simulink model "CW_m26"  (R2020b)
settings: Solver=ode3  StartTime=0.0  StopTime=simTime  FixedStep=0.001  RelTol=1e-3  EnableMultiTasking=on
undefined symbols (not defined in the file): b, J, K, L, R
settings Model: Creator=aarrieta  LastModifiedBy=Xiao Ling
settings DataIOCC: ExternalInput=var  SaveFormat=Array  SignalLogging=off  DSMLogging=off  ReturnWorkspaceOutputs=off
settings OptimizationCC: LifeSpan=inf
settings DebuggingCC: UnderspecifiedInitializationDetection=Classic  MergeDetectMultiDrivingBlocksExec=none  SolverPrmCheckMsg=warning  StateNameClashWarn=warning  SFUnexpectedBacktrackingDiag=warning  SFNoUnconditionalDefaultTransitionDiag=warning  SFExecutionAtInitializationDiag=none  ArithmeticOperatorsInVariantConditions=warning
settings HardwareCC: ProdBitPerPointer=32  ProdBitPerSizeT=32  ProdBitPerPtrDiffT=32  ProdLargestAtomicFloat=None  ProdIntDivRoundTo=Undefined  ProdEndianess=Unspecified  ProdWordSize=32  ProdHWDeviceType=32-bit Generic
settings ModelReferenceCC: PropagateSignalLabelsOutOfModel=off
settings SFSimCC: SimUseLocalCustomCode=off  CustomCodeUndefinedFunction=UseInterfaceOnly
settings RTWCC: RTWUseLocalCustomCode=off
settings CodeAppCC: StateflowObjectComments=on
settings GRTTargetCC: TargetLangStandard=C89/C90 (ANSI)
settings ConfigComp: CovScope=ReferencedModels  CovMetricSettings=dcmtw  CovHTMLOptions=-sRT=1 -aTS=1 -bRG=1 -bTC=1 -hTR=0 -nFC=0 -scm=1 -bcm=1 -xEv=0  CovSaveCumulativeToWorkspaceVar=on  CovSaveSingleToWorkspaceVar=on  DVMaxTestCaseSteps=500  DVTestSuiteOptimization=CombinedObjectives (Nonlinear Extended)  DVDetectActiveLogic=on
settings SimscapeCC: SimscapeNormalizeSystem=off
settings ConfigurationSet: Description=SimMechanics 2G

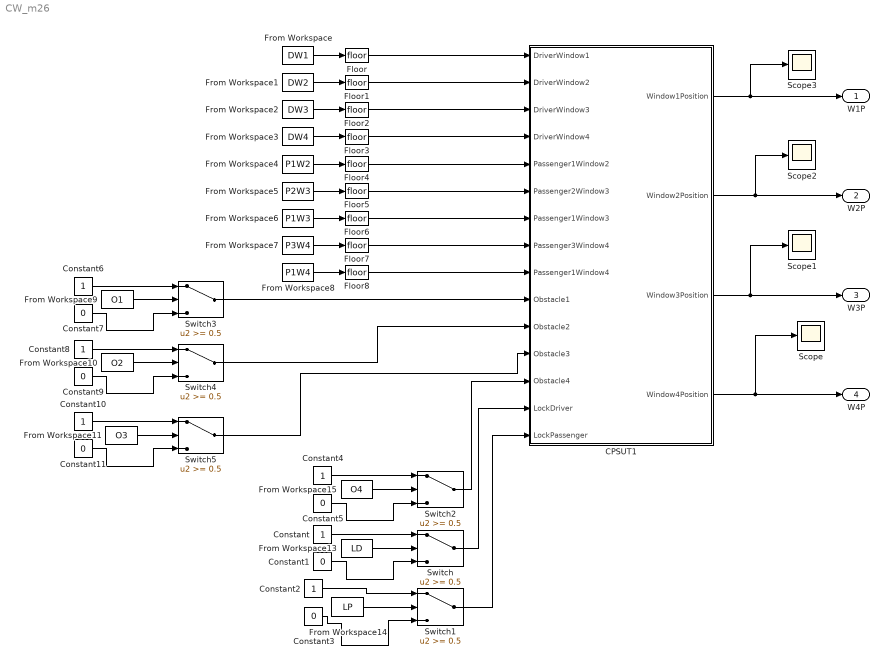
== system CW_m26 ==
  CPSUT1 : Subsystem
  Constant{,2,4,6,8,10} (6 alike) : Constant  OutDataTypeStr=boolean
  Constant{1,3,5,7,9,11} (6 alike) : Constant  Value=0  OutDataTypeStr=boolean
  Floor{,1..8} (9 alike) : Rounding
  From Workspace : FromWorkspace  VariableName=DW1
  From Workspace1 : FromWorkspace  VariableName=DW2
  From Workspace10 : FromWorkspace  VariableName=O2
  From Workspace11 : FromWorkspace  VariableName=O3
  From Workspace13 : FromWorkspace  VariableName=LD
  From Workspace14 : FromWorkspace  VariableName=LP
  From Workspace15 : FromWorkspace  VariableName=O4
  From Workspace2 : FromWorkspace  VariableName=DW3
  From Workspace3 : FromWorkspace  VariableName=DW4
  From Workspace4 : FromWorkspace  VariableName=P1W2
  From Workspace5 : FromWorkspace  VariableName=P2W3
  From Workspace6 : FromWorkspace  VariableName=P1W3
  From Workspace7 : FromWorkspace  VariableName=P3W4
  From Workspace8 : FromWorkspace  VariableName=P1W4
  From Workspace9 : FromWorkspace  VariableName=O1
  Scope{,1..3} (4 alike) : Scope
  Switch{,1..5} (6 alike) : Switch  Threshold=0.5
  W1P : Outport
  W2P : Outport  Port=2
  W3P : Outport  Port=3
  W4P : Outport  Port=4
  wires:
  CPSUT1/1(Window1Position) -> W1P/1, Scope3/1
  CPSUT1/2(Window2Position) -> W2P/1, Scope2/1
  CPSUT1/3(Window3Position) -> W3P/1, Scope1/1
  CPSUT1/4(Window4Position) -> W4P/1, Scope/1
  From Workspace2/1 -> Floor2/1
  From Workspace3/1 -> Floor3/1
  From Workspace4/1 -> Floor4/1
  From Workspace5/1 -> Floor5/1
  From Workspace6/1 -> Floor6/1
  From Workspace7/1 -> Floor7/1
  From Workspace8/1 -> Floor8/1
  Switch2/1 -> CPSUT1/13(Obstacle4)
  From Workspace13/1 -> Switch/2
  From Workspace14/1 -> Switch1/2
  Switch1/1 -> CPSUT1/15(LockPassenger)
  Constant/1 -> Switch/1
  Constant1/1 -> Switch/3
  Constant2/1 -> Switch1/1
  Constant3/1 -> Switch1/3
  Switch/1 -> CPSUT1/14(LockDriver)
  From Workspace/1 -> Floor/1
  Floor/1 -> CPSUT1/1(DriverWindow1)
  From Workspace1/1 -> Floor1/1
  Floor1/1 -> CPSUT1/2(DriverWindow2)
  Floor2/1 -> CPSUT1/3(DriverWindow3)
  Floor3/1 -> CPSUT1/4(DriverWindow4)
  Floor4/1 -> CPSUT1/5(Passenger1Window2)
  Floor5/1 -> CPSUT1/6(Passenger2Window3)
  Floor6/1 -> CPSUT1/7(Passenger1Window3)
  Floor7/1 -> CPSUT1/8(Passenger3Window4)
  Floor8/1 -> CPSUT1/9(Passenger1Window4)
  From Workspace15/1 -> Switch2/2
  Constant5/1 -> Switch2/3
  Constant4/1 -> Switch2/1
  Constant7/1 -> Switch3/3
  From Workspace9/1 -> Switch3/2
  Switch3/1 -> CPSUT1/10(Obstacle1)
  Constant6/1 -> Switch3/1
  Constant9/1 -> Switch4/3
  From Workspace10/1 -> Switch4/2
  Switch4/1 -> CPSUT1/11(Obstacle2)
  Constant8/1 -> Switch4/1
  Constant11/1 -> Switch5/3
  From Workspace11/1 -> Switch5/2
  Switch5/1 -> CPSUT1/12(Obstacle3)
  Constant10/1 -> Switch5/1

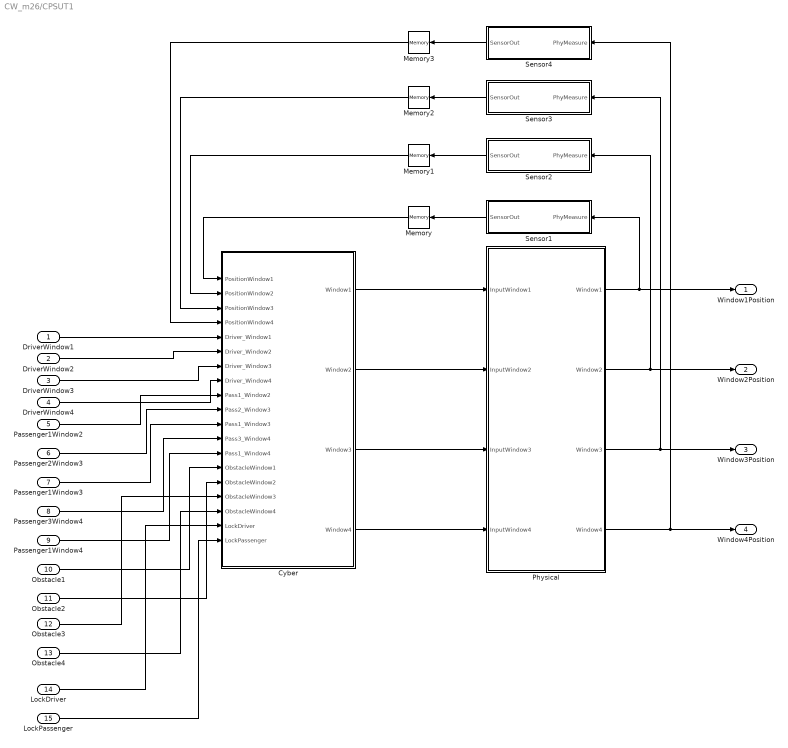
== system CW_m26/CPSUT1 ==
  DriverWindow1 : Inport
  DriverWindow2 : Inport  Port=2
  DriverWindow3 : Inport  Port=3
  DriverWindow4 : Inport  Port=4
  Passenger1Window2 : Inport  Port=5
  Passenger2Window3 : Inport  Port=6
  Passenger1Window3 : Inport  Port=7
  Passenger3Window4 : Inport  Port=8
  Passenger1Window4 : Inport  Port=9
  Obstacle1 : Inport  Port=10
  Obstacle2 : Inport  Port=11
  Obstacle3 : Inport  Port=12
  Obstacle4 : Inport  Port=13
  LockDriver : Inport  Port=14
  LockPassenger : Inport  Port=15
  Cyber : Subsystem
  Memory{,1..3} (4 alike) : Memory
  Physical : Subsystem
  Sensor1 : Subsystem
  Sensor2 : Subsystem
  Sensor3 : Subsystem
  Sensor4 : Subsystem
  Window1Position : Outport  VectorParamsAs1DForOutWhenUnconnected=off
  Window2Position : Outport  Port=2  VectorParamsAs1DForOutWhenUnconnected=off
  Window3Position : Outport  Port=3  VectorParamsAs1DForOutWhenUnconnected=off
  Window4Position : Outport  Port=4  VectorParamsAs1DForOutWhenUnconnected=off
  wires:
  Cyber/4(Window4) -> Physical/4(InputWindow4)
  Cyber/3(Window3) -> Physical/3(InputWindow3)
  Cyber/2(Window2) -> Physical/2(InputWindow2)
  Cyber/1(Window1) -> Physical/1(InputWindow1)
  Physical/1(Window1) -> Sensor1/1(PhyMeasure), Window1Position/1
  Physical/2(Window2) -> Sensor2/1(PhyMeasure), Window2Position/1
  Physical/3(Window3) -> Window3Position/1, Sensor3/1(PhyMeasure)
  Physical/4(Window4) -> Sensor4/1(PhyMeasure), Window4Position/1
  Memory/1 -> Cyber/1(PositionWindow1)
  Memory1/1 -> Cyber/2(PositionWindow2)
  Memory2/1 -> Cyber/3(PositionWindow3)
  Memory3/1 -> Cyber/4(PositionWindow4)
  Obstacle1/1 -> Cyber/14(ObstacleWindow1)
  Sensor4/1(SensorOut) -> Memory3/1
  Sensor3/1(SensorOut) -> Memory2/1
  Sensor2/1(SensorOut) -> Memory1/1
  Sensor1/1(SensorOut) -> Memory/1
  DriverWindow2/1 -> Cyber/6(Driver_Window2)
  DriverWindow1/1 -> Cyber/5(Driver_Window1)
  DriverWindow3/1 -> Cyber/7(Driver_Window3)
  DriverWindow4/1 -> Cyber/8(Driver_Window4)
  Passenger1Window2/1 -> Cyber/9(Pass1_Window2)
  Passenger2Window3/1 -> Cyber/10(Pass2_Window3)
  Passenger1Window3/1 -> Cyber/11(Pass1_Window3)
  Passenger3Window4/1 -> Cyber/12(Pass3_Window4)
  Passenger1Window4/1 -> Cyber/13(Pass1_Window4)
  Obstacle2/1 -> Cyber/15(ObstacleWindow2)
  Obstacle3/1 -> Cyber/16(ObstacleWindow3)
  Obstacle4/1 -> Cyber/17(ObstacleWindow4)
  LockDriver/1 -> Cyber/18(LockDriver)
  LockPassenger/1 -> Cyber/19(LockPassenger)

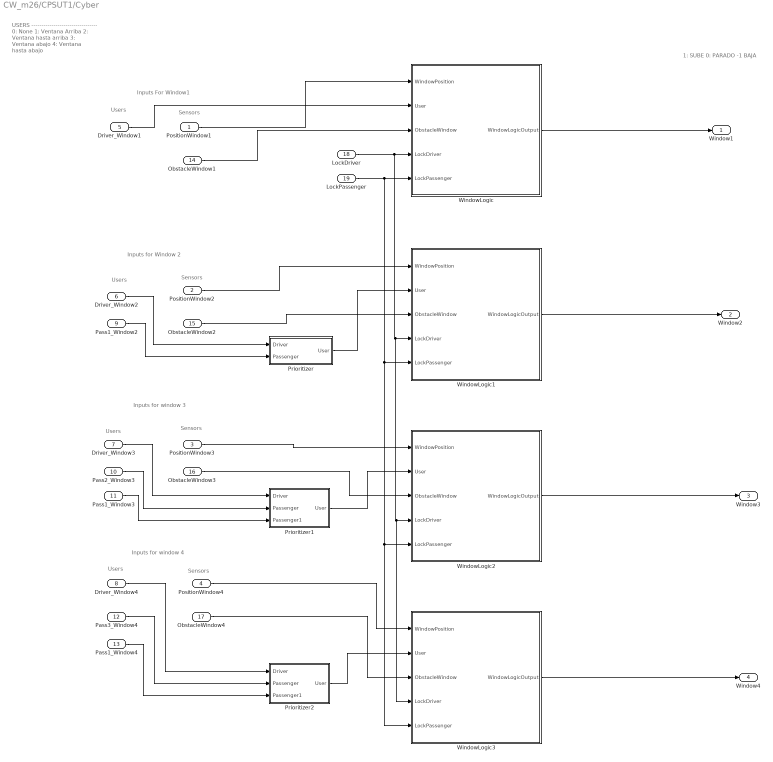
== system CW_m26/CPSUT1/Cyber ==
  note: 1: SUBE
      | 0: PARADO
      | -1 BAJA
  note: USERS
      | ---------------------------------
      | 0: None
      | 1: Ventana Arriba
      | 2: Ventana hasta arriba
      | 3: Ventana abajo
      | 4: Ventana hasta abajo
  note: Sensors
  note: Users
  note: Sensors
  note: Users
  note: Sensors
  note: Users
  note: Users
  note: Sensors
  note: Inputs for window 4
  note: Inputs for window 3
  note: Inputs for Window 2
  note: Inputs For Window1
  PositionWindow1 : Inport
  PositionWindow2 : Inport  Port=2
  PositionWindow3 : Inport  Port=3
  PositionWindow4 : Inport  Port=4
  Driver_Window1 : Inport  Port=5
  Driver_Window2 : Inport  Port=6
  Driver_Window3 : Inport  Port=7
  Driver_Window4 : Inport  Port=8
  Pass1_Window2 : Inport  Port=9
  Pass2_Window3 : Inport  Port=10
  Pass1_Window3 : Inport  Port=11
  Pass3_Window4 : Inport  Port=12
  Pass1_Window4 : Inport  Port=13
  ObstacleWindow1 : Inport  Port=14
  ObstacleWindow2 : Inport  Port=15
  ObstacleWindow3 : Inport  Port=16
  ObstacleWindow4 : Inport  Port=17
  LockDriver : Inport  Port=18
  LockPassenger : Inport  Port=19
  Prioritizer : Subsystem
  Prioritizer1 : Subsystem
  Prioritizer2 : Subsystem
  WindowLogic : Subsystem
  WindowLogic1 : Subsystem
  WindowLogic2 : Subsystem
  WindowLogic3 : Subsystem
  Window1 : Outport  VectorParamsAs1DForOutWhenUnconnected=off
  Window2 : Outport  Port=2  VectorParamsAs1DForOutWhenUnconnected=off
  Window3 : Outport  Port=3  VectorParamsAs1DForOutWhenUnconnected=off
  Window4 : Outport  Port=4  VectorParamsAs1DForOutWhenUnconnected=off
  wires:
  LockDriver/1 -> WindowLogic1/4(LockDriver), WindowLogic3/4(LockDriver), WindowLogic2/4(LockDriver), WindowLogic/4(LockDriver)
  LockPassenger/1 -> WindowLogic1/5(LockPassenger), WindowLogic3/5(LockPassenger), WindowLogic2/5(LockPassenger), WindowLogic/5(LockPassenger)
  PositionWindow1/1 -> WindowLogic/1(WindowPosition)
  ObstacleWindow1/1 -> WindowLogic/3(ObstacleWindow)
  Driver_Window1/1 -> WindowLogic/2(User)
  WindowLogic/1(WindowLogicOutput) -> Window1/1
  Prioritizer/1(User) -> WindowLogic1/2(User)
  Driver_Window2/1 -> Prioritizer/1(Driver)
  Pass1_Window2/1 -> Prioritizer/2(Passenger)
  PositionWindow2/1 -> WindowLogic1/1(WindowPosition)
  ObstacleWindow2/1 -> WindowLogic1/3(ObstacleWindow)
  WindowLogic1/1(WindowLogicOutput) -> Window2/1
  Prioritizer1/1(User) -> WindowLogic2/2(User)
  PositionWindow3/1 -> WindowLogic2/1(WindowPosition)
  ObstacleWindow3/1 -> WindowLogic2/3(ObstacleWindow)
  Driver_Window3/1 -> Prioritizer1/1(Driver)
  Pass2_Window3/1 -> Prioritizer1/2(Passenger)
  Pass1_Window3/1 -> Prioritizer1/3(Passenger1)
  Driver_Window4/1 -> Prioritizer2/1(Driver)
  Pass3_Window4/1 -> Prioritizer2/2(Passenger)
  Pass1_Window4/1 -> Prioritizer2/3(Passenger1)
  PositionWindow4/1 -> WindowLogic3/1(WindowPosition)
  ObstacleWindow4/1 -> WindowLogic3/3(ObstacleWindow)
  Prioritizer2/1(User) -> WindowLogic3/2(User)
  WindowLogic2/1(WindowLogicOutput) -> Window3/1
  WindowLogic3/1(WindowLogicOutput) -> Window4/1

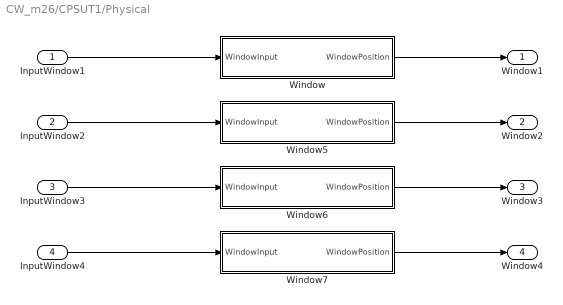
== system CW_m26/CPSUT1/Physical ==
  InputWindow1 : Inport
  InputWindow2 : Inport  Port=2
  InputWindow3 : Inport  Port=3
  InputWindow4 : Inport  Port=4
  Window : Subsystem
  Window5 : Subsystem
  Window6 : Subsystem
  Window7 : Subsystem
  Window1 : Outport  VectorParamsAs1DForOutWhenUnconnected=off
  Window2 : Outport  Port=2  VectorParamsAs1DForOutWhenUnconnected=off
  Window3 : Outport  Port=3  VectorParamsAs1DForOutWhenUnconnected=off
  Window4 : Outport  Port=4  VectorParamsAs1DForOutWhenUnconnected=off
  wires:
  InputWindow1/1 -> Window/1(WindowInput)
  InputWindow2/1 -> Window5/1(WindowInput)
  InputWindow3/1 -> Window6/1(WindowInput)
  InputWindow4/1 -> Window7/1(WindowInput)
  Window/1(WindowPosition) -> Window1/1
  Window5/1(WindowPosition) -> Window2/1
  Window6/1(WindowPosition) -> Window3/1
  Window7/1(WindowPosition) -> Window4/1

== system CW_m26/CPSUT1/Sensor1 ==
  PhyMeasure : Inport
  SensorOut : Outport  VectorParamsAs1DForOutWhenUnconnected=off
  wires:
  PhyMeasure/1 -> SensorOut/1

== system CW_m26/CPSUT1/Sensor2 ==
  PhyMeasure : Inport
  SensorOut : Outport  VectorParamsAs1DForOutWhenUnconnected=off
  wires:
  PhyMeasure/1 -> SensorOut/1

== system CW_m26/CPSUT1/Sensor3 ==
  PhyMeasure : Inport
  SensorOut : Outport  VectorParamsAs1DForOutWhenUnconnected=off
  wires:
  PhyMeasure/1 -> SensorOut/1

== system CW_m26/CPSUT1/Sensor4 ==
  PhyMeasure : Inport
  SensorOut : Outport  VectorParamsAs1DForOutWhenUnconnected=off
  wires:
  PhyMeasure/1 -> SensorOut/1

== system CW_m26/CPSUT1/Cyber/Prioritizer ==
  Driver : Inport
  Passenger : Inport  Port=2
  Switch : Switch  Criteria=u2 ~= 0
  User : Outport  VectorParamsAs1DForOutWhenUnconnected=off
  wires:
  Driver/1 -> Switch/1, Switch/2
  Passenger/1 -> Switch/3
  Switch/1 -> User/1

== system CW_m26/CPSUT1/Cyber/Prioritizer1 ==
  Driver : Inport
  Passenger : Inport  Port=2
  Passenger1 : Inport  Port=3
  Switch : Switch  Criteria=u2 ~= 0
  Switch1 : Switch  Criteria=u2 ~= 0
  User : Outport  VectorParamsAs1DForOutWhenUnconnected=off
  wires:
  Switch/1 -> User/1
  Passenger/1 -> Switch1/1, Switch1/2
  Driver/1 -> Switch/1, Switch/2
  Passenger1/1 -> Switch1/3
  Switch1/1 -> Switch/3

== system CW_m26/CPSUT1/Cyber/Prioritizer2 ==
  Driver : Inport
  Passenger : Inport  Port=2
  Passenger1 : Inport  Port=3
  Switch : Switch  Criteria=u2 ~= 0
  Switch1 : Switch  Criteria=u2 ~= 0
  User : Outport  VectorParamsAs1DForOutWhenUnconnected=off
  wires:
  Switch1/1 -> Switch/3
  Passenger1/1 -> Switch1/3
  Driver/1 -> Switch/2, Switch/1
  Passenger/1 -> Switch1/2, Switch1/1
  Switch/1 -> User/1

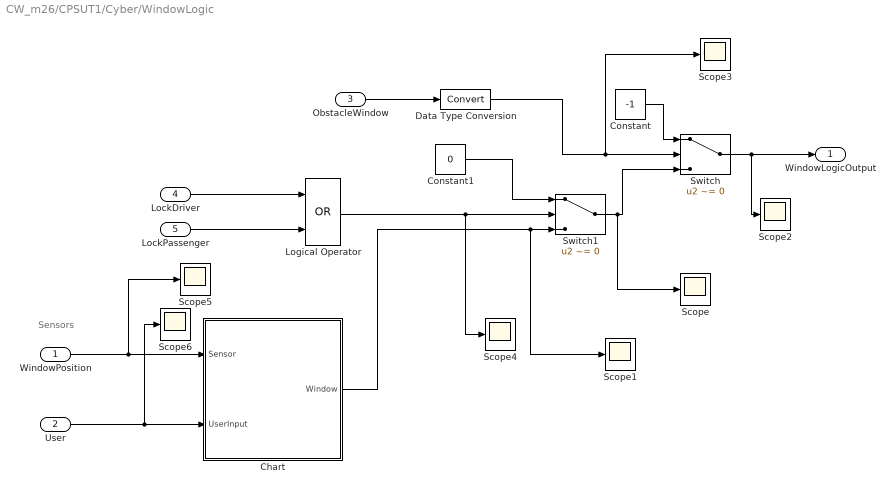
== system CW_m26/CPSUT1/Cyber/WindowLogic ==
  note: Sensors
  WindowPosition : Inport
  User : Inport  Port=2
  ObstacleWindow : Inport  Port=3
  LockDriver : Inport  Port=4
  LockPassenger : Inport  Port=5
  Chart : Stateflow chart  TreatAsAtomicUnit=on
  Constant : Constant  Value=-1
  Constant1 : Constant  Value=0
  Data Type Conversion : DataTypeConversion
  Logical Operator : Logic  Operator=OR  AllPortsSameDT=off  OutDataTypeStr=boolean
  Scope{,1..6} (7 alike) : Scope
  Switch : Switch  Criteria=u2 ~= 0  Threshold=1  ZeroCross=off
  Switch1 : Switch  Criteria=u2 ~= 0
  WindowLogicOutput : Outport  VectorParamsAs1DForOutWhenUnconnected=off
  wires:
  LockDriver/1 -> Logical Operator/1
  LockPassenger/1 -> Logical Operator/2
  ObstacleWindow/1 -> Data Type Conversion/1
  Switch/1 -> Scope2/1, WindowLogicOutput/1
  Constant1/1 -> Switch1/1
  Switch1/1 -> Scope/1, Switch/3
  WindowPosition/1 -> Scope5/1, Chart/1(Sensor)
  User/1 -> Chart/2(UserInput), Scope6/1
  Chart/1(Window) -> Scope1/1, Switch1/3
  Constant/1 -> Switch/1
  Data Type Conversion/1 -> Scope3/1, Switch/2
  Logical Operator/1 -> Scope4/1, Switch1/2

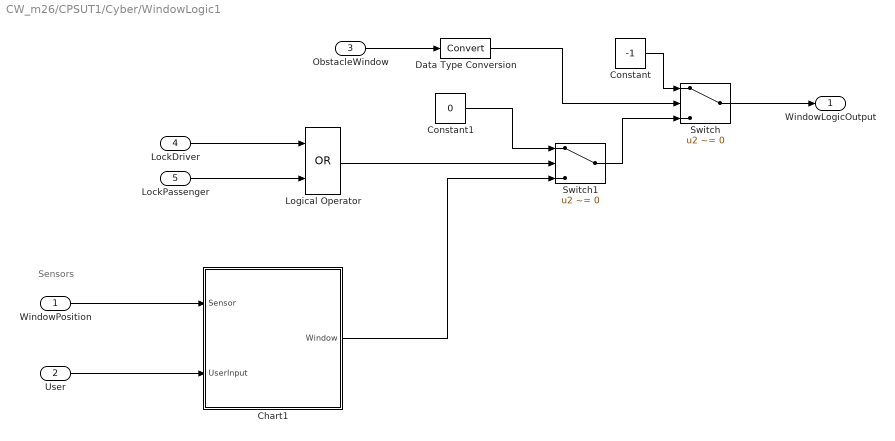
== system CW_m26/CPSUT1/Cyber/WindowLogic1 ==
  note: Sensors
  WindowPosition : Inport
  User : Inport  Port=2
  ObstacleWindow : Inport  Port=3
  LockDriver : Inport  Port=4
  LockPassenger : Inport  Port=5
  Chart1 : Stateflow chart  TreatAsAtomicUnit=on
  Constant : Constant  Value=-1
  Constant1 : Constant  Value=0
  Data Type Conversion : DataTypeConversion
  Logical Operator : Logic  Operator=OR  AllPortsSameDT=off  OutDataTypeStr=boolean
  Switch : Switch  Criteria=u2 ~= 0  Threshold=1  ZeroCross=off
  Switch1 : Switch  Criteria=u2 ~= 0
  WindowLogicOutput : Outport  VectorParamsAs1DForOutWhenUnconnected=off
  wires:
  Logical Operator/1 -> Switch1/2
  Data Type Conversion/1 -> Switch/2
  Constant/1 -> Switch/1
  Chart1/1(Window) -> Switch1/3
  User/1 -> Chart1/2(UserInput)
  WindowPosition/1 -> Chart1/1(Sensor)
  Switch1/1 -> Switch/3
  Constant1/1 -> Switch1/1
  Switch/1 -> WindowLogicOutput/1
  ObstacleWindow/1 -> Data Type Conversion/1
  LockPassenger/1 -> Logical Operator/2
  LockDriver/1 -> Logical Operator/1

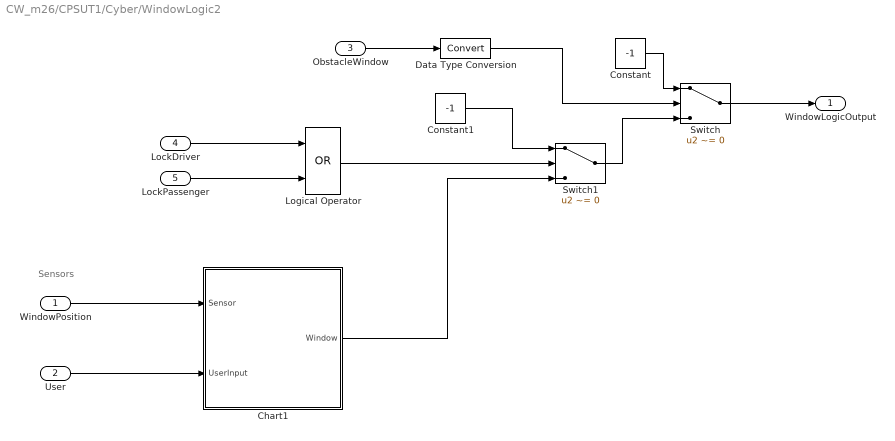
== system CW_m26/CPSUT1/Cyber/WindowLogic2 ==
  note: Sensors
  WindowPosition : Inport
  User : Inport  Port=2
  ObstacleWindow : Inport  Port=3
  LockDriver : Inport  Port=4
  LockPassenger : Inport  Port=5
  Chart1 : Stateflow chart  TreatAsAtomicUnit=on
  Constant : Constant  Value=-1
  Constant1 : Constant  Value=-1
  Data Type Conversion : DataTypeConversion
  Logical Operator : Logic  Operator=OR  AllPortsSameDT=off  OutDataTypeStr=boolean
  Switch : Switch  Criteria=u2 ~= 0  Threshold=1  ZeroCross=off
  Switch1 : Switch  Criteria=u2 ~= 0
  WindowLogicOutput : Outport  VectorParamsAs1DForOutWhenUnconnected=off
  wires:
  LockDriver/1 -> Logical Operator/1
  LockPassenger/1 -> Logical Operator/2
  ObstacleWindow/1 -> Data Type Conversion/1
  Switch/1 -> WindowLogicOutput/1
  Constant1/1 -> Switch1/1
  Switch1/1 -> Switch/3
  WindowPosition/1 -> Chart1/1(Sensor)
  User/1 -> Chart1/2(UserInput)
  Chart1/1(Window) -> Switch1/3
  Constant/1 -> Switch/1
  Data Type Conversion/1 -> Switch/2
  Logical Operator/1 -> Switch1/2

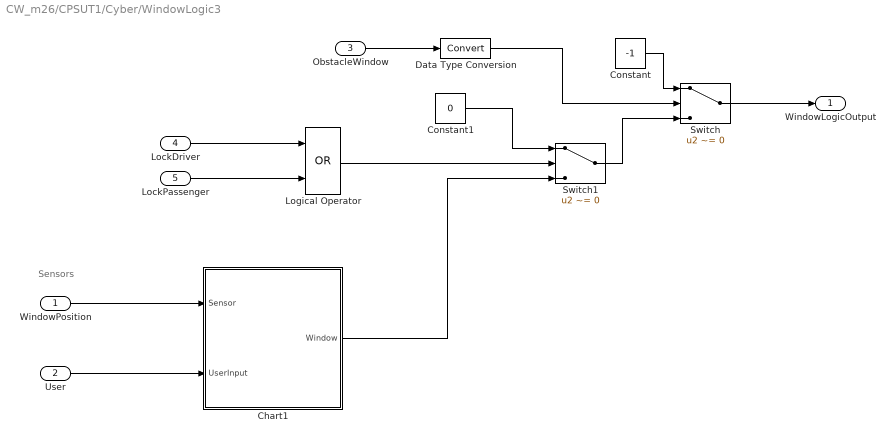
== system CW_m26/CPSUT1/Cyber/WindowLogic3 ==
  note: Sensors
  WindowPosition : Inport
  User : Inport  Port=2
  ObstacleWindow : Inport  Port=3
  LockDriver : Inport  Port=4
  LockPassenger : Inport  Port=5
  Chart1 : Stateflow chart  TreatAsAtomicUnit=on
  Constant : Constant  Value=-1
  Constant1 : Constant  Value=0
  Data Type Conversion : DataTypeConversion
  Logical Operator : Logic  Operator=OR  AllPortsSameDT=off  OutDataTypeStr=boolean
  Switch : Switch  Criteria=u2 ~= 0  Threshold=1  ZeroCross=off
  Switch1 : Switch  Criteria=u2 ~= 0
  WindowLogicOutput : Outport  VectorParamsAs1DForOutWhenUnconnected=off
  wires:
  Logical Operator/1 -> Switch1/2
  Data Type Conversion/1 -> Switch/2
  Constant/1 -> Switch/1
  Chart1/1(Window) -> Switch1/3
  User/1 -> Chart1/2(UserInput)
  WindowPosition/1 -> Chart1/1(Sensor)
  Switch1/1 -> Switch/3
  Constant1/1 -> Switch1/1
  Switch/1 -> WindowLogicOutput/1
  ObstacleWindow/1 -> Data Type Conversion/1
  LockPassenger/1 -> Logical Operator/2
  LockDriver/1 -> Logical Operator/1

== system CW_m26/CPSUT1/Physical/Window ==
  WindowInput : Inport
  DC_Engine : Subsystem
  Integrator : Integrator  InitialCondition=5  LimitOutput=on  UpperSaturationLimit=5  LowerSaturationLimit=0
  WindowPosition : Outport  VectorParamsAs1DForOutWhenUnconnected=off
  wires:
  Integrator/1 -> WindowPosition/1
  DC_Engine/1(Speed) -> Integrator/1
  WindowInput/1 -> DC_Engine/1(input)

== system CW_m26/CPSUT1/Physical/Window5 ==
  WindowInput : Inport
  DC_Engine : Subsystem
  Integrator : Integrator  InitialCondition=5  LimitOutput=on  UpperSaturationLimit=5  LowerSaturationLimit=0
  WindowPosition : Outport  VectorParamsAs1DForOutWhenUnconnected=off
  wires:
  WindowInput/1 -> DC_Engine/1(input)
  DC_Engine/1(Speed) -> Integrator/1
  Integrator/1 -> WindowPosition/1

== system CW_m26/CPSUT1/Physical/Window6 ==
  WindowInput : Inport
  DC_Engine : Subsystem
  Integrator : Integrator  InitialCondition=5  LimitOutput=on  UpperSaturationLimit=5  LowerSaturationLimit=0
  WindowPosition : Outport  VectorParamsAs1DForOutWhenUnconnected=off
  wires:
  Integrator/1 -> WindowPosition/1
  DC_Engine/1(Speed) -> Integrator/1
  WindowInput/1 -> DC_Engine/1(input)

== system CW_m26/CPSUT1/Physical/Window7 ==
  WindowInput : Inport
  DC_Engine : Subsystem
  Integrator : Integrator  InitialCondition=5  LimitOutput=on  UpperSaturationLimit=5  LowerSaturationLimit=0
  WindowPosition : Outport  VectorParamsAs1DForOutWhenUnconnected=off
  wires:
  WindowInput/1 -> DC_Engine/1(input)
  DC_Engine/1(Speed) -> Integrator/1
  Integrator/1 -> WindowPosition/1

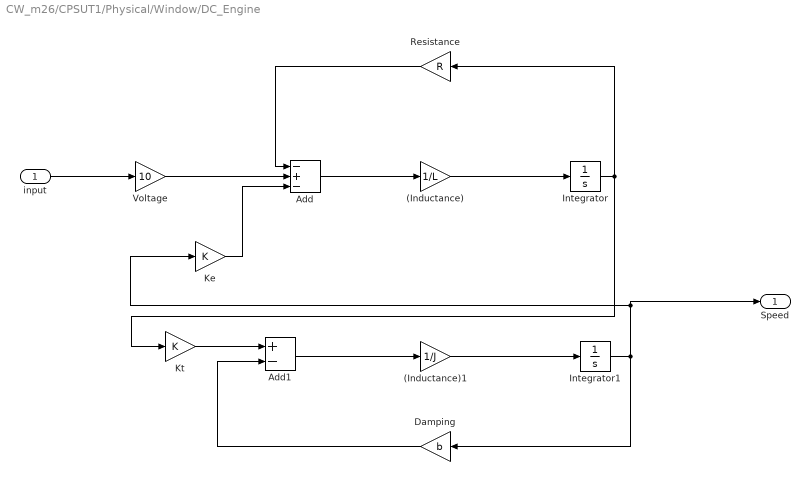
== system CW_m26/CPSUT1/Physical/Window/DC_Engine ==
  input : Inport
  (Inductance) : Gain  Gain=1/L
  (Inductance)1 : Gain  Gain=1/J
  Add : Sum  Inputs=-+-
  Add1 : Sum  Inputs=+-
  Damping : Gain  Gain=b
  Integrator : Integrator
  Integrator1 : Integrator
  Ke : Gain  Gain=K
  Kt : Gain  Gain=K
  Resistance : Gain  Gain=R
  Voltage : Gain  Gain=10
  Speed : Outport  VectorParamsAs1DForOutWhenUnconnected=off
  wires:
  input/1 -> Voltage/1
  Voltage/1 -> Add/2
  Add/1 -> (Inductance)/1
  (Inductance)/1 -> Integrator/1
  Integrator/1 -> Kt/1, Resistance/1
  Resistance/1 -> Add/1
  Ke/1 -> Add/3
  Kt/1 -> Add1/1
  Add1/1 -> (Inductance)1/1
  (Inductance)1/1 -> Integrator1/1
  Integrator1/1 -> Ke/1, Speed/1, Damping/1
  Damping/1 -> Add1/2

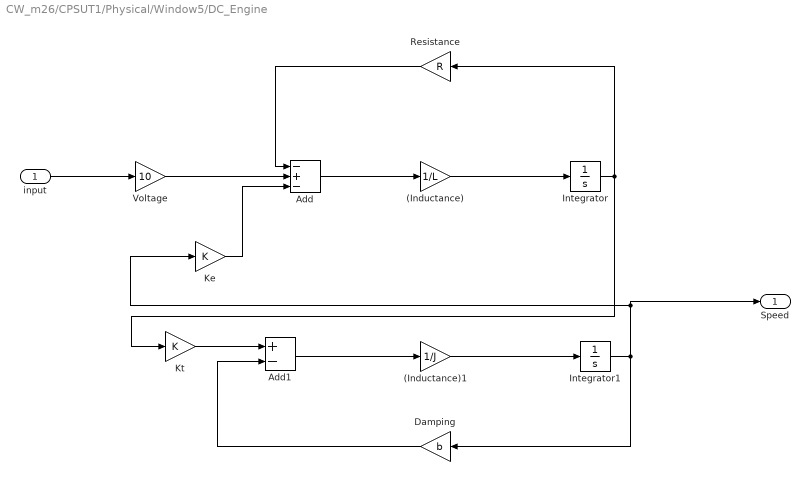
== system CW_m26/CPSUT1/Physical/Window5/DC_Engine ==
  input : Inport
  (Inductance) : Gain  Gain=1/L
  (Inductance)1 : Gain  Gain=1/J
  Add : Sum  Inputs=-+-
  Add1 : Sum  Inputs=+-
  Damping : Gain  Gain=b
  Integrator : Integrator
  Integrator1 : Integrator
  Ke : Gain  Gain=K
  Kt : Gain  Gain=K
  Resistance : Gain  Gain=R
  Voltage : Gain  Gain=10
  Speed : Outport  VectorParamsAs1DForOutWhenUnconnected=off
  wires:
  Damping/1 -> Add1/2
  Integrator1/1 -> Damping/1, Speed/1, Ke/1
  (Inductance)1/1 -> Integrator1/1
  Add1/1 -> (Inductance)1/1
  Kt/1 -> Add1/1
  Ke/1 -> Add/3
  Resistance/1 -> Add/1
  Integrator/1 -> Resistance/1, Kt/1
  (Inductance)/1 -> Integrator/1
  Add/1 -> (Inductance)/1
  Voltage/1 -> Add/2
  input/1 -> Voltage/1

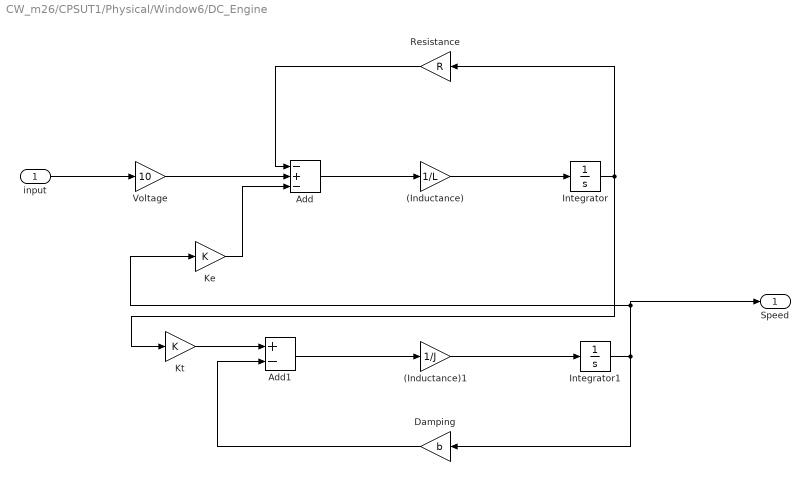
== system CW_m26/CPSUT1/Physical/Window6/DC_Engine ==
  input : Inport
  (Inductance) : Gain  Gain=1/L
  (Inductance)1 : Gain  Gain=1/J
  Add : Sum  Inputs=-+-
  Add1 : Sum  Inputs=+-
  Damping : Gain  Gain=b
  Integrator : Integrator
  Integrator1 : Integrator
  Ke : Gain  Gain=K
  Kt : Gain  Gain=K
  Resistance : Gain  Gain=R
  Voltage : Gain  Gain=10
  Speed : Outport  VectorParamsAs1DForOutWhenUnconnected=off
  wires:
  input/1 -> Voltage/1
  Voltage/1 -> Add/2
  Add/1 -> (Inductance)/1
  (Inductance)/1 -> Integrator/1
  Integrator/1 -> Kt/1, Resistance/1
  Resistance/1 -> Add/1
  Ke/1 -> Add/3
  Kt/1 -> Add1/1
  Add1/1 -> (Inductance)1/1
  (Inductance)1/1 -> Integrator1/1
  Integrator1/1 -> Ke/1, Speed/1, Damping/1
  Damping/1 -> Add1/2

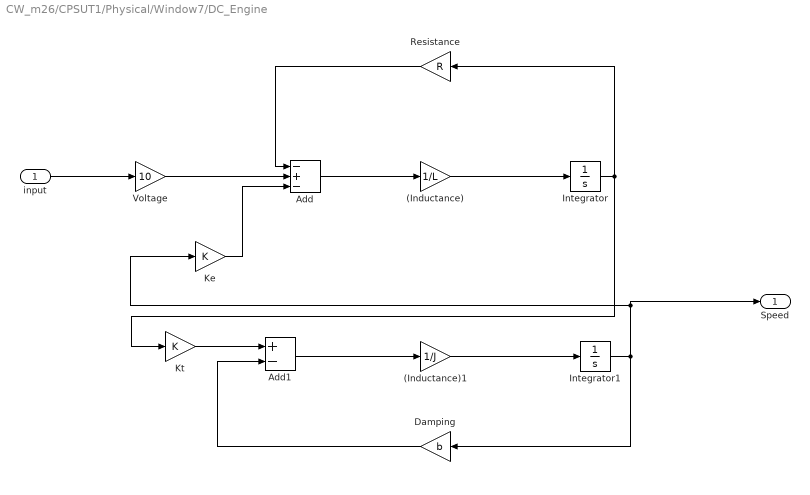
== system CW_m26/CPSUT1/Physical/Window7/DC_Engine ==
  input : Inport
  (Inductance) : Gain  Gain=1/L
  (Inductance)1 : Gain  Gain=1/J
  Add : Sum  Inputs=-+-
  Add1 : Sum  Inputs=+-
  Damping : Gain  Gain=b
  Integrator : Integrator
  Integrator1 : Integrator
  Ke : Gain  Gain=K
  Kt : Gain  Gain=K
  Resistance : Gain  Gain=R
  Voltage : Gain  Gain=10
  Speed : Outport  VectorParamsAs1DForOutWhenUnconnected=off
  wires:
  Damping/1 -> Add1/2
  Integrator1/1 -> Damping/1, Speed/1, Ke/1
  (Inductance)1/1 -> Integrator1/1
  Add1/1 -> (Inductance)1/1
  Kt/1 -> Add1/1
  Ke/1 -> Add/3
  Resistance/1 -> Add/1
  Integrator/1 -> Resistance/1, Kt/1
  (Inductance)/1 -> Integrator/1
  Add/1 -> (Inductance)/1
  Voltage/1 -> Add/2
  input/1 -> Voltage/1

== stateflow chart CW_m26/CPSUT1/Cyber/WindowLogic1/Chart1 ==
  state Bajand_hasta_abajo
    entry: Window = -1;
  state Bajando
    entry: Window = -1;
  state Idle
    entry:Window = 0;
  state Subiendo_hasta_arriba
    entry: Window = 1;
  state Subiendo
    entry: Window = 1;
  Subiendo -> Bajand_hasta_abajo [order 4] : [UserInput==4]
  Bajand_hasta_abajo -> Bajando [order 2] : [UserInput==3]
  Subiendo -> Bajando [order 3] : [UserInput==3]
  Bajando -> Bajand_hasta_abajo [order 2] : [UserInput==4]
  Idle -> Bajando [order 3] : [UserInput==3&&Sensor>0]
  Subiendo_hasta_arriba -> Bajand_hasta_abajo [order 3] : [UserInput==4]
  Idle -> Bajand_hasta_abajo [order 4] : [UserInput==4&&Sensor>0]
  Bajando -> Subiendo [order 3] : [UserInput==1]
  Subiendo_hasta_arriba -> Bajando [order 4] : [UserInput==3]
  Bajand_hasta_abajo -> Subiendo [order 4] : [UserInput==1]
  Bajand_hasta_abajo -> Idle [order 1] : [Sensor<=0]
  Bajand_hasta_abajo -> Subiendo_hasta_arriba [order 3] : [UserInput==2]
  Bajando -> Idle [order 1] : [Sensor<=0||UserInput==0]
  Bajando -> Subiendo_hasta_arriba [order 4] : [UserInput==2]
  (default) -> Idle
  Idle -> Subiendo_hasta_arriba [order 2] : [UserInput==2&&Sensor<5]
  Idle -> Subiendo [order 1] : [UserInput == 1&&Sensor<5]
  Subiendo -> Idle [order 1] : [Sensor>=5||UserInput==0]
  Subiendo_hasta_arriba -> Idle [order 1] : [Sensor >=5]
  Subiendo_hasta_arriba -> Subiendo [order 2] : [UserInput ==1]
  Subiendo -> Subiendo_hasta_arriba [order 2] : [UserInput==2]
  data: Sensor input; UserInput input; Window output double

== stateflow chart CW_m26/CPSUT1/Cyber/WindowLogic/Chart ==
  state Bajand_hasta_abajo
    entry: Window = -1;
  state Bajando
    entry: Window = -1;
  state Idle
    entry:Window = 0;
  state Subiendo_hasta_arriba
    entry: Window = 1;
  state Subiendo
    entry: Window = 1;
  Subiendo -> Bajand_hasta_abajo [order 4] : [UserInput==4]
  Bajand_hasta_abajo -> Bajando [order 2] : [UserInput==3]
  Subiendo -> Bajando [order 3] : [UserInput==3]
  Bajando -> Bajand_hasta_abajo [order 2] : [UserInput==4]
  Idle -> Bajando [order 3] : [UserInput==3&&Sensor>0]
  Subiendo_hasta_arriba -> Bajand_hasta_abajo [order 3] : [UserInput==4]
  Idle -> Bajand_hasta_abajo [order 4] : [UserInput==4&&Sensor>0]
  Bajando -> Subiendo [order 3] : [UserInput==1]
  Subiendo_hasta_arriba -> Bajando [order 4] : [UserInput==3]
  Bajand_hasta_abajo -> Subiendo [order 4] : [UserInput==1]
  Bajand_hasta_abajo -> Idle [order 1] : [Sensor<=0]
  Bajand_hasta_abajo -> Subiendo_hasta_arriba [order 3] : [UserInput==2]
  Bajando -> Idle [order 1] : [Sensor<=0||UserInput==0]
  Bajando -> Subiendo_hasta_arriba [order 4] : [UserInput==2]
  (default) -> Idle
  Idle -> Subiendo_hasta_arriba [order 2] : [UserInput==2&&Sensor<5]
  Idle -> Subiendo [order 1] : [UserInput == 1&&Sensor<5]
  Subiendo -> Idle [order 1] : [Sensor>=5||UserInput==0]
  Subiendo_hasta_arriba -> Idle [order 1] : [Sensor >=5]
  Subiendo_hasta_arriba -> Subiendo [order 2] : [UserInput ==1]
  Subiendo -> Subiendo_hasta_arriba [order 2] : [UserInput==2]
  data: Sensor input; UserInput input; Window output double

== stateflow chart CW_m26/CPSUT1/Cyber/WindowLogic2/Chart1 ==
  state Bajand_hasta_abajo
    entry: Window = -1;
  state Bajando
    entry: Window = -1;
  state Idle
    entry:Window = 0;
  state Subiendo_hasta_arriba
    entry: Window = 1;
  state Subiendo
    entry: Window = 1;
  Subiendo -> Bajand_hasta_abajo [order 4] : [UserInput==4]
  Bajand_hasta_abajo -> Bajando [order 2] : [UserInput==3]
  Subiendo -> Bajando [order 3] : [UserInput==3]
  Bajando -> Bajand_hasta_abajo [order 2] : [UserInput==4]
  Idle -> Bajando [order 3] : [UserInput==3&&Sensor>0]
  Subiendo_hasta_arriba -> Bajand_hasta_abajo [order 3] : [UserInput==4]
  Idle -> Bajand_hasta_abajo [order 4] : [UserInput==4&&Sensor>0]
  Bajando -> Subiendo [order 3] : [UserInput==1]
  Subiendo_hasta_arriba -> Bajando [order 4] : [UserInput==3]
  Bajand_hasta_abajo -> Subiendo [order 4] : [UserInput==1]
  Bajand_hasta_abajo -> Idle [order 1] : [Sensor<=0]
  Bajand_hasta_abajo -> Subiendo_hasta_arriba [order 3] : [UserInput==2]
  Bajando -> Idle [order 1] : [Sensor<=0||UserInput==0]
  Bajando -> Subiendo_hasta_arriba [order 4] : [UserInput==2]
  (default) -> Idle
  Idle -> Subiendo_hasta_arriba [order 2] : [UserInput==2&&Sensor<5]
  Idle -> Subiendo [order 1] : [UserInput == 1&&Sensor<5]
  Subiendo -> Idle [order 1] : [Sensor>=5||UserInput==0]
  Subiendo_hasta_arriba -> Idle [order 1] : [Sensor >=5]
  Subiendo_hasta_arriba -> Subiendo [order 2] : [UserInput ==1]
  Subiendo -> Subiendo_hasta_arriba [order 2] : [UserInput==2]
  data: Sensor input; UserInput input; Window output double

== stateflow chart CW_m26/CPSUT1/Cyber/WindowLogic3/Chart1 ==
  state Bajand_hasta_abajo
    entry: Window = -1;
  state Bajando
    entry: Window = -1;
  state Idle
    entry:Window = 0;
  state Subiendo_hasta_arriba
    entry: Window = 1;
  state Subiendo
    entry: Window = 1;
  Subiendo -> Bajand_hasta_abajo [order 4] : [UserInput==4]
  Bajand_hasta_abajo -> Bajando [order 2] : [UserInput==3]
  Subiendo -> Bajando [order 3] : [UserInput==3]
  Bajando -> Bajand_hasta_abajo [order 2] : [UserInput==4]
  Idle -> Bajando [order 3] : [UserInput==3&&Sensor>0]
  Subiendo_hasta_arriba -> Bajand_hasta_abajo [order 3] : [UserInput==4]
  Idle -> Bajand_hasta_abajo [order 4] : [UserInput==4&&Sensor>0]
  Bajando -> Subiendo [order 3] : [UserInput==1]
  Subiendo_hasta_arriba -> Bajando [order 4] : [UserInput==3]
  Bajand_hasta_abajo -> Subiendo [order 4] : [UserInput==1]
  Bajand_hasta_abajo -> Idle [order 1] : [Sensor<=0]
  Bajand_hasta_abajo -> Subiendo_hasta_arriba [order 3] : [UserInput==2]
  Bajando -> Idle [order 1] : [Sensor<=0||UserInput==0]
  Bajando -> Subiendo_hasta_arriba [order 4] : [UserInput==2]
  (default) -> Idle
  Idle -> Subiendo_hasta_arriba [order 2] : [UserInput==2&&Sensor<5]
  Idle -> Subiendo [order 1] : [UserInput == 1&&Sensor<5]
  Subiendo -> Idle [order 1] : [Sensor>=5||UserInput==0]
  Subiendo_hasta_arriba -> Idle [order 1] : [Sensor >=5]
  Subiendo_hasta_arriba -> Subiendo [order 2] : [UserInput ==1]
  Subiendo -> Subiendo_hasta_arriba [order 2] : [UserInput==2]
  data: Sensor input; UserInput input; Window output double
